simulink model "main_controller"  (R2017a)
settings: Solver=VariableStepAuto  StartTime=0.0  StopTime=10.0  RelTol=1e-3
settings Model: Creator=Vincent  LastModifiedBy=Vincent

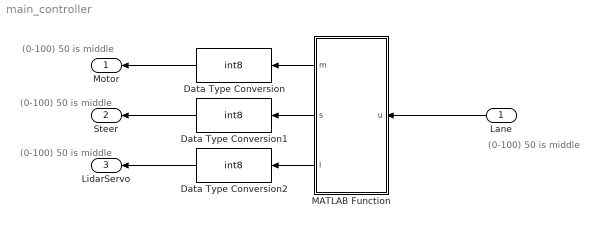
== system main_controller ==
  note: (0-100)
      | 50 is middle
  note: (0-100)
      | 50 is middle
  note: (0-100)
      | 50 is middle
  note: (0-100)
      | 50 is middle
  Lane : Inport
  Data Type Conversion : DataTypeConversion  OutDataTypeStr=int8
  Data Type Conversion1 : DataTypeConversion  OutDataTypeStr=int8
  Data Type Conversion2 : DataTypeConversion  OutDataTypeStr=int8
  MATLAB Function : MATLAB Function  TreatAsAtomicUnit=on
  Motor : Outport
  Steer : Outport  Port=2
  "LidarServo " : Outport  Port=3
  wires:
  Data Type Conversion/1 -> Motor/1
  Data Type Conversion1/1 -> Steer/1
  Data Type Conversion2/1 -> "LidarServo "/1
  Lane/1 -> MATLAB Function/1(u)
  MATLAB Function/1(m) -> Data Type Conversion/1
  MATLAB Function/2(s) -> Data Type Conversion1/1
  MATLAB Function/3(l) -> Data Type Conversion2/1

== matlab function main_controller/MATLAB Function ==
  data: u input; m output; s output; l output
function [m, s, l]= fcn(u)
    if(u == 50)
        m = 75;
    elseif(u >= 0 && u < 50)
        k = 50-u;
        m = 75-(k/3);
    elseif(u > 50 && u < 100)
        k = u-50;
        m = 75-(k/3);
    else
        m = 0;
    end
    s = -u
    l = u
end
